simulink model "Lab14Simulink"  (R2021b)
settings: Solver=VariableStepAuto  StartTime=0.0  StopTime=0.05  RelTol=1e-3
undefined symbols (not defined in the file or in its folder): Bf, J, Ke, Kpwm, Kt, La, Ra
settings Model: Creator=User  LastModifiedBy=User

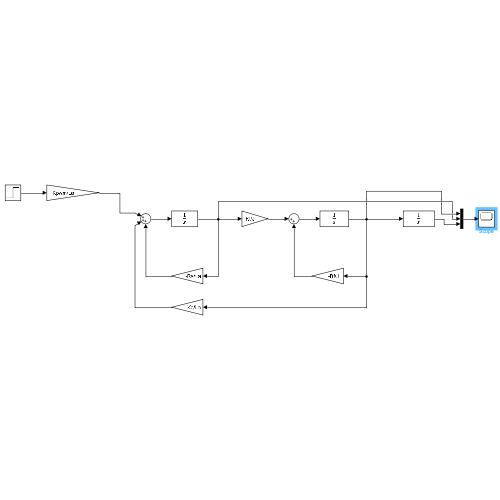
[thumbnail: Simulink's stored preview of the top-level diagram]
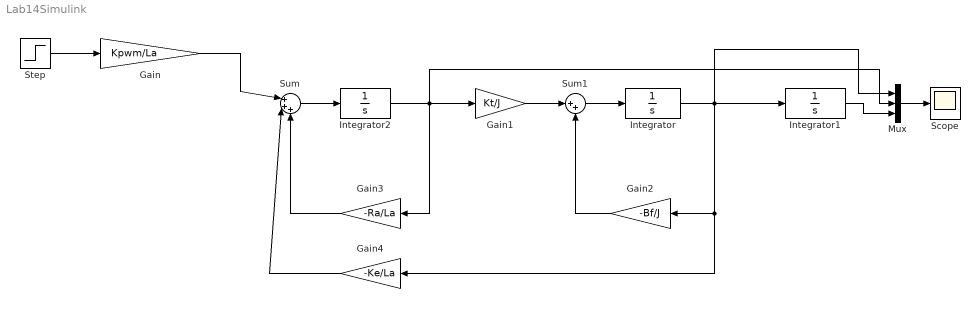
== system Lab14Simulink ==
  Gain : Gain  Gain=Kpwm/La
  Gain1 : Gain  Gain=Kt/J
  Gain2 : Gain  Gain=-Bf/J
  Gain3 : Gain  Gain=-Ra/La
  Gain4 : Gain  Gain=-Ke/La
  Integrator : Integrator
  Integrator1 : Integrator
  Integrator2 : Integrator
  Mux : Mux  Inputs=3
  Scope : Scope
  Step : Step  Time=0  SampleTime=0
  Sum : Sum  Inputs=|+++
  Sum1 : Sum  Inputs=|++
  wires:
  Step/1 -> Gain/1
  Gain1/1 -> Sum1/1
  Sum1/1 -> Integrator/1
  Integrator/1 -> Integrator1/1, Mux/1, Gain4/1, Gain2/1
  Gain2/1 -> Sum1/2
  Gain3/1 -> Sum/3
  Gain4/1 -> Sum/2
  Gain/1 -> Sum/1
  Mux/1 -> Scope/1
  Integrator1/1 -> Mux/3
  Sum/1 -> Integrator2/1
  Integrator2/1 -> Mux/2, Gain3/1, Gain1/1
